simulink model "PoliArd_calibration_2015a"  (R2015a)
settings: Solver=ode3  StartTime=0.0  StopTime=inf  FixedStep=0.001  RelTol=1e-3
values from neighbouring files (symbols this model uses):
  b = 0.025    [Main_PoliArd_calibration.m]
  cx = polyfit(out_scopex,hx,1)    [Main_PoliArd_calibration.m]    (also in calibration.mat = [1.83578189847e-05 0.000815203238403])
  cy = polyfit(out_scopey,hy,1)    [Main_PoliArd_calibration.m]    (also in calibration.mat = [1.80605123685e-05 -0.00194285103796])
libraries: PoliArd x12
settings Model: CovHtmlReporting=off  ExtModeTrigDuration=2  Creator=User  LastModifiedBy=User
settings OptimizationCC: LifeSpan=1
settings DebuggingCC: UnderspecifiedInitializationDetection=Classic  MergeDetectMultiDrivingBlocksExec=none
settings HardwareCC: ProdLargestAtomicInteger=Long  ProdLargestAtomicFloat=Double  ProdEndianess=LittleEndian  ProdHWDeviceType=ARM Compatible->ARM Cortex
settings RTWCC: SystemTargetFile=realtime.tlc  GenerateMakefile=off  TemplateMakefile=realtime.tmf  Description=Run on Target Hardware  RTWVerbose=off
settings ERTTargetCC: CombineOutputUpdateFcns=off  ExtModeTransport=3  ExtModeMexFile=ext_serial_win32_comm_rtt  ExtModeMexArgs=0 1 9600  InlinedParameterPlacement=Hierarchical  ERTSrcFileBannerTemplate=realtime_code_template.cgt  ERTHdrFileBannerTemplate=realtime_code_template.cgt  ERTDataSrcFileTemplate=realtime_code_template.cgt  ERTDataHdrFileTemplate=realtime_code_template.cgt  ERTCustomFileTemplate=realtime_file_process.tlc

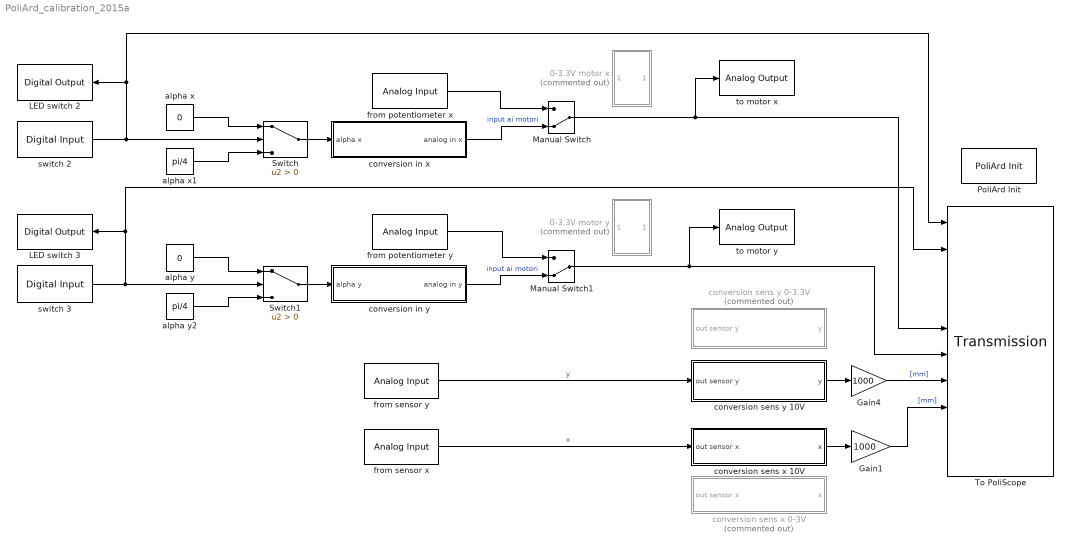
== system PoliArd_calibration_2015a ==
  0-3.3V motor x : Subsystem  Commented=on
  "0-3.3V motor y " : Subsystem  Commented=on
  Gain1 : Gain  Gain=1000
  Gain4 : Gain  Gain=1000
  "LED switch 2 " : PoliArd/Digital Output  DO_pin=1
  "LED switch 3 " : PoliArd/Digital Output  DO_pin=2
  Manual Switch : ManualSwitch  CurrentSetting=0
  Manual Switch1 : ManualSwitch  CurrentSetting=0
  PoliArd Init : PoliArd/PoliArd Init
  Switch : Switch  Criteria=u2 > Threshold
  Switch1 : Switch  Criteria=u2 > Threshold
  To PoliScope : PoliArd/Transmission  sample_freq=1000  sig_to_send=6
  alpha x : Constant  Value=0
  alpha x1 : Constant  Value=pi/4
  alpha y : Constant  Value=0
  alpha y2 : Constant  Value=pi/4
  conversion in x : Subsystem
  conversion in y : Subsystem
  conversion sens x 0-3V : Subsystem  Commented=on
  conversion sens x 10V : Subsystem
  conversion sens y 0-3.3V : Subsystem  Commented=on
  conversion sens y 10V : Subsystem
  from potentiometer x : PoliArd/Analog Input  AIpin_mask=8  AIsample=-1
  from potentiometer y : PoliArd/Analog Input  AIpin_mask=9  AIsample=-1
  from sensor x : PoliArd/Analog Input  AIpin_mask=4  AIsample=-1
  from sensor y : PoliArd/Analog Input  AIpin_mask=3  AIsample=-1
  switch 2 : PoliArd/Digital Input  DI_pin=2  DIsample=-1
  switch 3 : PoliArd/Digital Input  DI_pin=3  DIsample=-1
  to motor x : PoliArd/Analog Output  DAC_pin_mask=1
  to motor y : PoliArd/Analog Output  DAC_pin_mask=2
  wires:
  conversion in x/1(analog in x) -> Manual Switch/2  "input ai motori"
  from potentiometer x/1 -> Manual Switch/1
  from potentiometer y/1 -> Manual Switch1/1
  conversion in y/1(analog in y) -> Manual Switch1/2  "input ai motori"
  Manual Switch/1 -> To PoliScope/5, to motor x/1
  Manual Switch1/1 -> To PoliScope/6, to motor y/1
  from sensor x/1 -> conversion sens x 10V/1(out sensor x)  "x"
  from sensor y/1 -> conversion sens y 10V/1(out sensor y)  "y"
  conversion sens x 10V/1(x) -> Gain1/1
  conversion sens y 10V/1(y) -> Gain4/1
  Gain1/1 -> To PoliScope/8  "[mm]"
  Gain4/1 -> To PoliScope/7  "[mm]"
  Switch/1 -> conversion in x/1(alpha x)
  Switch1/1 -> conversion in y/1(alpha y)
  alpha x/1 -> Switch/1
  alpha x1/1 -> Switch/3
  switch 2/1 -> "LED switch 2 "/1, To PoliScope/1, Switch/2
  alpha y/1 -> Switch1/1
  alpha y2/1 -> Switch1/3
  switch 3/1 -> "LED switch 3 "/1, To PoliScope/2, Switch1/2

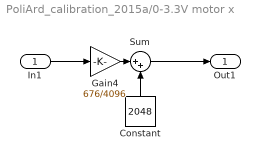
== system PoliArd_calibration_2015a/0-3.3V motor x ==
  In1 : Inport
  Constant : Constant  Value=2048
  Gain4 : Gain  Gain=676/4096
  Sum : Sum  Inputs=|++
  Out1 : Outport
  wires:
  Sum/1 -> Out1/1
  Gain4/1 -> Sum/1
  Constant/1 -> Sum/2
  In1/1 -> Gain4/1

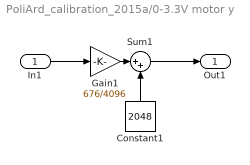
== system PoliArd_calibration_2015a/0-3.3V motor y  ==
  In1 : Inport
  Constant1 : Constant  Value=2048
  Gain1 : Gain  Gain=676/4096
  Sum1 : Sum  Inputs=|++
  Out1 : Outport
  wires:
  Sum1/1 -> Out1/1
  Gain1/1 -> Sum1/1
  Constant1/1 -> Sum1/2
  In1/1 -> Gain1/1

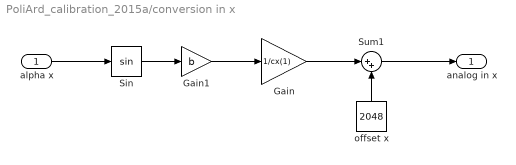
== system PoliArd_calibration_2015a/conversion in x ==
  alpha x : Inport
  Gain : Gain  Gain=1/cx(1)
  Gain1 : Gain  Gain=b
  Sin : Trigonometry
  Sum1 : Sum  Inputs=|++
  offset x : Constant  Value=2048
  analog in x : Outport
  wires:
  alpha x/1 -> Sin/1
  offset x/1 -> Sum1/2
  Sum1/1 -> analog in x/1
  Gain/1 -> Sum1/1
  Gain1/1 -> Gain/1
  Sin/1 -> Gain1/1

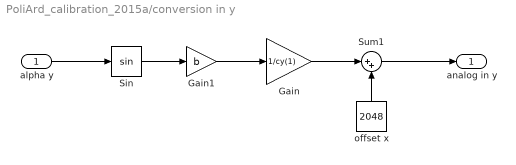
== system PoliArd_calibration_2015a/conversion in y ==
  alpha y : Inport
  Gain : Gain  Gain=1/cy(1)
  Gain1 : Gain  Gain=b
  Sin : Trigonometry
  Sum1 : Sum  Inputs=|++
  offset x : Constant  Value=2048
  analog in y : Outport
  wires:
  Sin/1 -> Gain1/1
  Gain1/1 -> Gain/1
  Gain/1 -> Sum1/1
  Sum1/1 -> analog in y/1
  offset x/1 -> Sum1/2
  alpha y/1 -> Sin/1

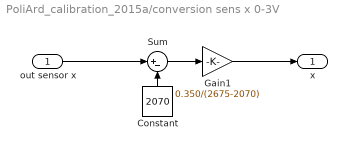
== system PoliArd_calibration_2015a/conversion sens x 0-3V ==
  out sensor x : Inport
  Constant : Constant  Value=2070
  Gain1 : Gain  Gain=0.350/(2675-2070)
  Sum : Sum  Inputs=|+-
  x : Outport
  wires:
  Constant/1 -> Sum/2
  Sum/1 -> Gain1/1
  out sensor x/1 -> Sum/1
  Gain1/1 -> x/1

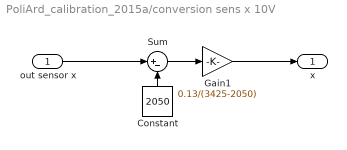
== system PoliArd_calibration_2015a/conversion sens x 10V ==
  out sensor x : Inport
  Constant : Constant  Value=2050
  Gain1 : Gain  Gain=0.13/(3425-2050)
  Sum : Sum  Inputs=|+-
  x : Outport
  wires:
  Gain1/1 -> x/1
  out sensor x/1 -> Sum/1
  Sum/1 -> Gain1/1
  Constant/1 -> Sum/2

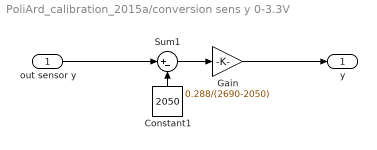
== system PoliArd_calibration_2015a/conversion sens y 0-3.3V ==
  out sensor y : Inport
  Constant1 : Constant  Value=2050
  Gain : Gain  Gain=0.288/(2690-2050)
  Sum1 : Sum  Inputs=|+-
  y : Outport
  wires:
  out sensor y/1 -> Sum1/1
  Sum1/1 -> Gain/1
  Constant1/1 -> Sum1/2
  Gain/1 -> y/1

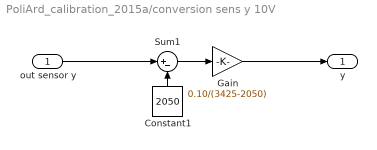
== system PoliArd_calibration_2015a/conversion sens y 10V ==
  out sensor y : Inport
  Constant1 : Constant  Value=2050
  Gain : Gain  Gain=0.10/(3425-2050)
  Sum1 : Sum  Inputs=|+-
  y : Outport
  wires:
  Gain/1 -> y/1
  Constant1/1 -> Sum1/2
  Sum1/1 -> Gain/1
  out sensor y/1 -> Sum1/1
